simulink model "IFSSIM_Brakes"  (R2025b)
settings: Solver=FixedStepDiscrete  StartTime=0  StopTime=inf  FixedStep=1/960  RelTol=1e-3
settings Model: Creator=raulmoran  LastModifiedBy=raulmoran

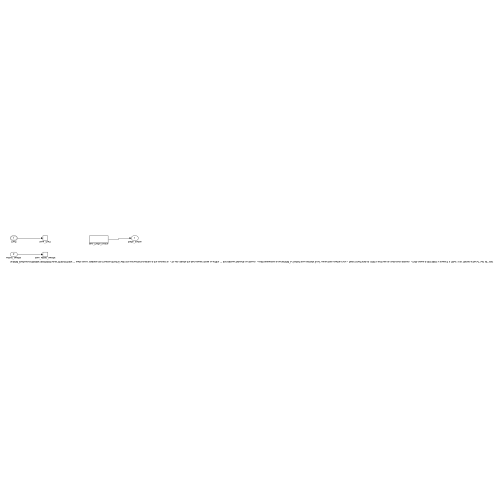
[thumbnail: Simulink's stored preview of the top-level diagram]
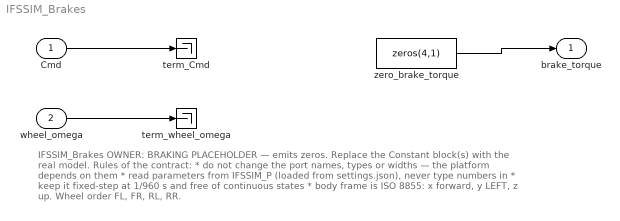
== system IFSSIM_Brakes ==
  note: IFSSIM_Brakes\n\nOWNER: BRAKING\n\nPLACEHOLDER — emits zeros. Replace the Constant block(s) with the real model.\n\nRules of the contract:\n * do not change the port names, types or widths — the platform depends on them\n * read parameters from IFSSIM_P (loaded from settings.json), never type numbers in\n * keep it fixed-step at 1/960 s and free of continuous states\n * body frame is ISO 8855: x forward, y LEFT, z up. Wheel order FL, FR, RL, RR.
  Cmd : Inport  OutDataTypeStr=Bus: IFSSIM_CmdBus  BusOutputAsStruct=on
  wheel_omega : Inport  Port=2  PortDimensions=4
  term_Cmd : Terminator
  term_wheel_omega : Terminator
  zero_brake_torque : Constant  Value=zeros(4,1)
  brake_torque : Outport  PortDimensions=4
  wires:
  Cmd/1 -> term_Cmd/1
  wheel_omega/1 -> term_wheel_omega/1
  zero_brake_torque/1 -> brake_torque/1
